simulink model "sist_noise_comp"  (Simulink 7.2)
settings: Solver=ode45  StartTime=0.0  StopTime=10  RelTol=1e-3
libraries: simulink_extras x1
settings Model: Creator=CrisGC  LastModifiedBy=CrisGC

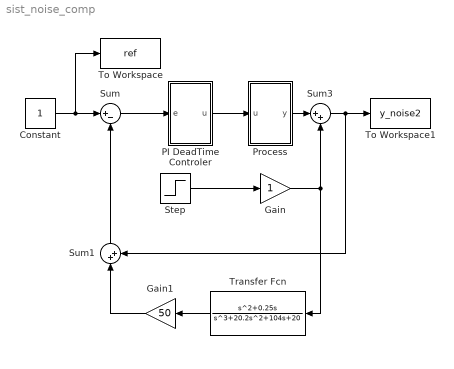
== system sist_noise_comp ==
  Constant : Constant  OutDataType=sfix(16)  OutScaling=2^0
  Gain : Gain  ParameterDataType=sfix(16)  ParameterScaling=2^0  OutDataType=sfix(16)  OutScaling=2^0
  Gain1 : Gain  Orientation=left  Gain=50  ParameterDataType=sfix(16)  ParameterScaling=2^0  OutDataType=sfix(16)  OutScaling=2^0
  PI DeadTime Controler : Subsystem
  Process : Subsystem
  Step : Step  Time=5  SampleTime=0
  Sum : Sum  Inputs=|+-  OutDataType=sfix(16)  OutScaling=2^0
  Sum1 : Sum  Orientation=up  Inputs=|++  OutDataType=sfix(16)  OutScaling=2^0
  Sum3 : Sum  Inputs=|++  OutDataType=sfix(16)  OutScaling=2^0
  To Workspace : ToWorkspace  VariableName=ref  SampleTime=-1  SaveFormat=Array
  To Workspace1 : ToWorkspace  VariableName=y_noise2  SampleTime=-1  SaveFormat=Array
  Transfer Fcn : TransferFcn  Orientation=left  Numerator=[1 0.25 0]  Denominator=[1 20.2 104 20]
  wires:
  Constant/1 -> Sum/1, To Workspace/1
  Sum/1 -> PI DeadTime Controler/1(e)
  Process/1(y) -> Sum3/1
  PI DeadTime Controler/1(u) -> Process/1(u)
  Gain/1 -> Sum3/2, Transfer Fcn/1
  Sum3/1 -> Sum1/2, To Workspace1/1
  Step/1 -> Gain/1
  Sum1/1 -> Sum/2
  Gain1/1 -> Sum1/1
  Transfer Fcn/1 -> Gain1/1

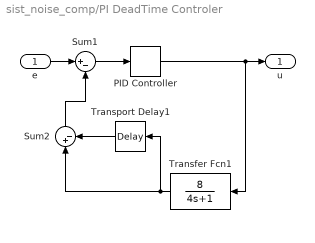
== system sist_noise_comp/PI DeadTime Controler ==
  e : Inport
  PID Controller : simulink_extras/Additional Linear/PID Controller  SystemSampleTime=-1  P=1  I=0.2  D=0
  Sum1 : Sum  Inputs=|+-  OutDataType=sfix(16)  OutScaling=2^0
  Sum2 : Sum  Orientation=up  Inputs=|+-  OutDataType=sfix(16)  OutScaling=2^0
  Transfer Fcn1 : TransferFcn  Orientation=left  Numerator=[8]  Denominator=[4 1]
  Transport Delay1 : TransportDelay  Orientation=left
  u : Outport
  wires:
  e/1 -> Sum1/1
  Sum2/1 -> Sum1/2
  Transport Delay1/1 -> Sum2/2
  Transfer Fcn1/1 -> Sum2/1, Transport Delay1/1
  Sum1/1 -> PID Controller/1
  PID Controller/1 -> u/1, Transfer Fcn1/1

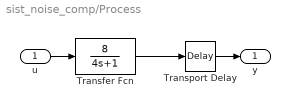
== system sist_noise_comp/Process ==
  u : Inport
  Transfer Fcn : TransferFcn  Numerator=[8]  Denominator=[4 1]
  Transport Delay : TransportDelay
  y : Outport
  wires:
  Transport Delay/1 -> y/1
  u/1 -> Transfer Fcn/1
  Transfer Fcn/1 -> Transport Delay/1
